simulink model "cic_filter_testing_8"  (Simulink 7.4)
settings: Solver=ode45  StartTime=0.0  StopTime=10000  RelTol=1e-3
undefined symbols (not defined in the file or in its folder): xlRetrieveParam
libraries: xbsIndex_r4 x441
(part 3 of 3)

== system cic_filter_testing_8/Parallel_CIC_filter1/Stage1_dec2/int_2/adder_tree7 ==
  sync : Inport
  din_1 : Inport  Port=2
  din_2 : Inport  Port=3
  din_3 : Inport  Port=4
  din_4 : Inport  Port=5
  din_5 : Inport  Port=6
  din_6 : Inport  Port=7
  din_7 : Inport  Port=8
  din_8 : Inport  Port=9
  adder_{0..6} (7 alike) : xbsIndex_r4/AddSub  mode=Addition  use_carryin=off  use_carryout=off  en=off  latency=1  precision=Full  arith_type=Unsigned  n_bits=18  bin_pt=17  quantization="Round  (unbiased: +/- Inf)"  overflow=Wrap  dbl_ovrd=off  use_behavioral_HDL=on  hw_selection=Fabric  pipelined=off  block_type=addsub
  sync_delay : xbsIndex_r4/Delay  en=off  latency=3  dbl_ovrd=off  reg_retiming=off  block_type=delay
      settings: block_version=11.4
  sync_out : Outport
  dout : Outport  Port=2
  wires:
  adder_6/1 -> dout/1
  adder_4/1 -> adder_6/2
  adder_5/1 -> adder_6/1
  adder_2/1 -> adder_5/2
  adder_3/1 -> adder_5/1
  adder_0/1 -> adder_4/2
  adder_1/1 -> adder_4/1
  din_7/1 -> adder_3/2
  din_8/1 -> adder_3/1
  din_5/1 -> adder_2/2
  din_6/1 -> adder_2/1
  din_3/1 -> adder_1/2
  din_4/1 -> adder_1/1
  din_1/1 -> adder_0/2
  din_2/1 -> adder_0/1
  sync_delay/1 -> sync_out/1
  sync/1 -> sync_delay/1

== system cic_filter_testing_8/Parallel_CIC_filter1/Stage1_dec2/int_2/adder_tree8 ==
  sync : Inport
  din_1 : Inport  Port=2
  din_2 : Inport  Port=3
  din_3 : Inport  Port=4
  din_4 : Inport  Port=5
  din_5 : Inport  Port=6
  din_6 : Inport  Port=7
  din_7 : Inport  Port=8
  din_8 : Inport  Port=9
  adder_{0..6} (7 alike) : xbsIndex_r4/AddSub  mode=Addition  use_carryin=off  use_carryout=off  en=off  latency=1  precision=Full  arith_type=Unsigned  n_bits=18  bin_pt=17  quantization="Round  (unbiased: +/- Inf)"  overflow=Wrap  dbl_ovrd=off  use_behavioral_HDL=on  hw_selection=Fabric  pipelined=off  block_type=addsub
  sync_delay : xbsIndex_r4/Delay  en=off  latency=3  dbl_ovrd=off  reg_retiming=off  block_type=delay
      settings: block_version=11.4
  sync_out : Outport
  dout : Outport  Port=2
  wires:
  adder_6/1 -> dout/1
  adder_4/1 -> adder_6/2
  adder_5/1 -> adder_6/1
  adder_2/1 -> adder_5/2
  adder_3/1 -> adder_5/1
  adder_0/1 -> adder_4/2
  adder_1/1 -> adder_4/1
  din_7/1 -> adder_3/2
  din_8/1 -> adder_3/1
  din_5/1 -> adder_2/2
  din_6/1 -> adder_2/1
  din_3/1 -> adder_1/2
  din_4/1 -> adder_1/1
  din_1/1 -> adder_0/2
  din_2/1 -> adder_0/1
  sync_delay/1 -> sync_out/1
  sync/1 -> sync_delay/1

== system cic_filter_testing_8/Parallel_CIC_filter1/Stage1_dec2/int_3/adder_tree1 ==
  sync : Inport
  din_1 : Inport  Port=2
  din_2 : Inport  Port=3
  din_3 : Inport  Port=4
  din_4 : Inport  Port=5
  din_5 : Inport  Port=6
  din_6 : Inport  Port=7
  din_7 : Inport  Port=8
  din_8 : Inport  Port=9
  adder_{0..6} (7 alike) : xbsIndex_r4/AddSub  mode=Addition  use_carryin=off  use_carryout=off  en=off  latency=1  precision=Full  arith_type=Unsigned  n_bits=18  bin_pt=17  quantization="Round  (unbiased: +/- Inf)"  overflow=Wrap  dbl_ovrd=off  use_behavioral_HDL=on  hw_selection=Fabric  pipelined=off  block_type=addsub
  sync_delay : xbsIndex_r4/Delay  en=off  latency=3  dbl_ovrd=off  reg_retiming=off  block_type=delay
      settings: block_version=11.4
  sync_out : Outport
  dout : Outport  Port=2
  wires:
  adder_6/1 -> dout/1
  adder_4/1 -> adder_6/2
  adder_5/1 -> adder_6/1
  adder_2/1 -> adder_5/2
  adder_3/1 -> adder_5/1
  adder_0/1 -> adder_4/2
  adder_1/1 -> adder_4/1
  din_7/1 -> adder_3/2
  din_8/1 -> adder_3/1
  din_5/1 -> adder_2/2
  din_6/1 -> adder_2/1
  din_3/1 -> adder_1/2
  din_4/1 -> adder_1/1
  din_1/1 -> adder_0/2
  din_2/1 -> adder_0/1
  sync_delay/1 -> sync_out/1
  sync/1 -> sync_delay/1

== system cic_filter_testing_8/Parallel_CIC_filter1/Stage1_dec2/int_3/adder_tree2 ==
  sync : Inport
  din_1 : Inport  Port=2
  din_2 : Inport  Port=3
  din_3 : Inport  Port=4
  din_4 : Inport  Port=5
  din_5 : Inport  Port=6
  din_6 : Inport  Port=7
  din_7 : Inport  Port=8
  din_8 : Inport  Port=9
  adder_{0..6} (7 alike) : xbsIndex_r4/AddSub  mode=Addition  use_carryin=off  use_carryout=off  en=off  latency=1  precision=Full  arith_type=Unsigned  n_bits=18  bin_pt=17  quantization="Round  (unbiased: +/- Inf)"  overflow=Wrap  dbl_ovrd=off  use_behavioral_HDL=on  hw_selection=Fabric  pipelined=off  block_type=addsub
  sync_delay : xbsIndex_r4/Delay  en=off  latency=3  dbl_ovrd=off  reg_retiming=off  block_type=delay
      settings: block_version=11.4
  sync_out : Outport
  dout : Outport  Port=2
  wires:
  adder_6/1 -> dout/1
  adder_4/1 -> adder_6/2
  adder_5/1 -> adder_6/1
  adder_2/1 -> adder_5/2
  adder_3/1 -> adder_5/1
  adder_0/1 -> adder_4/2
  adder_1/1 -> adder_4/1
  din_7/1 -> adder_3/2
  din_8/1 -> adder_3/1
  din_5/1 -> adder_2/2
  din_6/1 -> adder_2/1
  din_3/1 -> adder_1/2
  din_4/1 -> adder_1/1
  din_1/1 -> adder_0/2
  din_2/1 -> adder_0/1
  sync_delay/1 -> sync_out/1
  sync/1 -> sync_delay/1

== system cic_filter_testing_8/Parallel_CIC_filter1/Stage1_dec2/int_3/adder_tree3 ==
  sync : Inport
  din_1 : Inport  Port=2
  din_2 : Inport  Port=3
  din_3 : Inport  Port=4
  din_4 : Inport  Port=5
  din_5 : Inport  Port=6
  din_6 : Inport  Port=7
  din_7 : Inport  Port=8
  din_8 : Inport  Port=9
  adder_{0..6} (7 alike) : xbsIndex_r4/AddSub  mode=Addition  use_carryin=off  use_carryout=off  en=off  latency=1  precision=Full  arith_type=Unsigned  n_bits=18  bin_pt=17  quantization="Round  (unbiased: +/- Inf)"  overflow=Wrap  dbl_ovrd=off  use_behavioral_HDL=on  hw_selection=Fabric  pipelined=off  block_type=addsub
  sync_delay : xbsIndex_r4/Delay  en=off  latency=3  dbl_ovrd=off  reg_retiming=off  block_type=delay
      settings: block_version=11.4
  sync_out : Outport
  dout : Outport  Port=2
  wires:
  adder_6/1 -> dout/1
  adder_4/1 -> adder_6/2
  adder_5/1 -> adder_6/1
  adder_2/1 -> adder_5/2
  adder_3/1 -> adder_5/1
  adder_0/1 -> adder_4/2
  adder_1/1 -> adder_4/1
  din_7/1 -> adder_3/2
  din_8/1 -> adder_3/1
  din_5/1 -> adder_2/2
  din_6/1 -> adder_2/1
  din_3/1 -> adder_1/2
  din_4/1 -> adder_1/1
  din_1/1 -> adder_0/2
  din_2/1 -> adder_0/1
  sync_delay/1 -> sync_out/1
  sync/1 -> sync_delay/1

== system cic_filter_testing_8/Parallel_CIC_filter1/Stage1_dec2/int_3/adder_tree4 ==
  sync : Inport
  din_1 : Inport  Port=2
  din_2 : Inport  Port=3
  din_3 : Inport  Port=4
  din_4 : Inport  Port=5
  din_5 : Inport  Port=6
  din_6 : Inport  Port=7
  din_7 : Inport  Port=8
  din_8 : Inport  Port=9
  adder_{0..6} (7 alike) : xbsIndex_r4/AddSub  mode=Addition  use_carryin=off  use_carryout=off  en=off  latency=1  precision=Full  arith_type=Unsigned  n_bits=18  bin_pt=17  quantization="Round  (unbiased: +/- Inf)"  overflow=Wrap  dbl_ovrd=off  use_behavioral_HDL=on  hw_selection=Fabric  pipelined=off  block_type=addsub
  sync_delay : xbsIndex_r4/Delay  en=off  latency=3  dbl_ovrd=off  reg_retiming=off  block_type=delay
      settings: block_version=11.4
  sync_out : Outport
  dout : Outport  Port=2
  wires:
  adder_6/1 -> dout/1
  adder_4/1 -> adder_6/2
  adder_5/1 -> adder_6/1
  adder_2/1 -> adder_5/2
  adder_3/1 -> adder_5/1
  adder_0/1 -> adder_4/2
  adder_1/1 -> adder_4/1
  din_7/1 -> adder_3/2
  din_8/1 -> adder_3/1
  din_5/1 -> adder_2/2
  din_6/1 -> adder_2/1
  din_3/1 -> adder_1/2
  din_4/1 -> adder_1/1
  din_1/1 -> adder_0/2
  din_2/1 -> adder_0/1
  sync_delay/1 -> sync_out/1
  sync/1 -> sync_delay/1

== system cic_filter_testing_8/Parallel_CIC_filter1/Stage1_dec2/int_3/adder_tree5 ==
  sync : Inport
  din_1 : Inport  Port=2
  din_2 : Inport  Port=3
  din_3 : Inport  Port=4
  din_4 : Inport  Port=5
  din_5 : Inport  Port=6
  din_6 : Inport  Port=7
  din_7 : Inport  Port=8
  din_8 : Inport  Port=9
  adder_{0..6} (7 alike) : xbsIndex_r4/AddSub  mode=Addition  use_carryin=off  use_carryout=off  en=off  latency=1  precision=Full  arith_type=Unsigned  n_bits=18  bin_pt=17  quantization="Round  (unbiased: +/- Inf)"  overflow=Wrap  dbl_ovrd=off  use_behavioral_HDL=on  hw_selection=Fabric  pipelined=off  block_type=addsub
  sync_delay : xbsIndex_r4/Delay  en=off  latency=3  dbl_ovrd=off  reg_retiming=off  block_type=delay
      settings: block_version=11.4
  sync_out : Outport
  dout : Outport  Port=2
  wires:
  adder_6/1 -> dout/1
  adder_4/1 -> adder_6/2
  adder_5/1 -> adder_6/1
  adder_2/1 -> adder_5/2
  adder_3/1 -> adder_5/1
  adder_0/1 -> adder_4/2
  adder_1/1 -> adder_4/1
  din_7/1 -> adder_3/2
  din_8/1 -> adder_3/1
  din_5/1 -> adder_2/2
  din_6/1 -> adder_2/1
  din_3/1 -> adder_1/2
  din_4/1 -> adder_1/1
  din_1/1 -> adder_0/2
  din_2/1 -> adder_0/1
  sync_delay/1 -> sync_out/1
  sync/1 -> sync_delay/1

== system cic_filter_testing_8/Parallel_CIC_filter1/Stage1_dec2/int_3/adder_tree6 ==
  sync : Inport
  din_1 : Inport  Port=2
  din_2 : Inport  Port=3
  din_3 : Inport  Port=4
  din_4 : Inport  Port=5
  din_5 : Inport  Port=6
  din_6 : Inport  Port=7
  din_7 : Inport  Port=8
  din_8 : Inport  Port=9
  adder_{0..6} (7 alike) : xbsIndex_r4/AddSub  mode=Addition  use_carryin=off  use_carryout=off  en=off  latency=1  precision=Full  arith_type=Unsigned  n_bits=18  bin_pt=17  quantization="Round  (unbiased: +/- Inf)"  overflow=Wrap  dbl_ovrd=off  use_behavioral_HDL=on  hw_selection=Fabric  pipelined=off  block_type=addsub
  sync_delay : xbsIndex_r4/Delay  en=off  latency=3  dbl_ovrd=off  reg_retiming=off  block_type=delay
      settings: block_version=11.4
  sync_out : Outport
  dout : Outport  Port=2
  wires:
  adder_6/1 -> dout/1
  adder_4/1 -> adder_6/2
  adder_5/1 -> adder_6/1
  adder_2/1 -> adder_5/2
  adder_3/1 -> adder_5/1
  adder_0/1 -> adder_4/2
  adder_1/1 -> adder_4/1
  din_7/1 -> adder_3/2
  din_8/1 -> adder_3/1
  din_5/1 -> adder_2/2
  din_6/1 -> adder_2/1
  din_3/1 -> adder_1/2
  din_4/1 -> adder_1/1
  din_1/1 -> adder_0/2
  din_2/1 -> adder_0/1
  sync_delay/1 -> sync_out/1
  sync/1 -> sync_delay/1

== system cic_filter_testing_8/Parallel_CIC_filter1/Stage1_dec2/int_3/adder_tree7 ==
  sync : Inport
  din_1 : Inport  Port=2
  din_2 : Inport  Port=3
  din_3 : Inport  Port=4
  din_4 : Inport  Port=5
  din_5 : Inport  Port=6
  din_6 : Inport  Port=7
  din_7 : Inport  Port=8
  din_8 : Inport  Port=9
  adder_{0..6} (7 alike) : xbsIndex_r4/AddSub  mode=Addition  use_carryin=off  use_carryout=off  en=off  latency=1  precision=Full  arith_type=Unsigned  n_bits=18  bin_pt=17  quantization="Round  (unbiased: +/- Inf)"  overflow=Wrap  dbl_ovrd=off  use_behavioral_HDL=on  hw_selection=Fabric  pipelined=off  block_type=addsub
  sync_delay : xbsIndex_r4/Delay  en=off  latency=3  dbl_ovrd=off  reg_retiming=off  block_type=delay
      settings: block_version=11.4
  sync_out : Outport
  dout : Outport  Port=2
  wires:
  adder_6/1 -> dout/1
  adder_4/1 -> adder_6/2
  adder_5/1 -> adder_6/1
  adder_2/1 -> adder_5/2
  adder_3/1 -> adder_5/1
  adder_0/1 -> adder_4/2
  adder_1/1 -> adder_4/1
  din_7/1 -> adder_3/2
  din_8/1 -> adder_3/1
  din_5/1 -> adder_2/2
  din_6/1 -> adder_2/1
  din_3/1 -> adder_1/2
  din_4/1 -> adder_1/1
  din_1/1 -> adder_0/2
  din_2/1 -> adder_0/1
  sync_delay/1 -> sync_out/1
  sync/1 -> sync_delay/1

== system cic_filter_testing_8/Parallel_CIC_filter1/Stage1_dec2/int_3/adder_tree8 ==
  sync : Inport
  din_1 : Inport  Port=2
  din_2 : Inport  Port=3
  din_3 : Inport  Port=4
  din_4 : Inport  Port=5
  din_5 : Inport  Port=6
  din_6 : Inport  Port=7
  din_7 : Inport  Port=8
  din_8 : Inport  Port=9
  adder_{0..6} (7 alike) : xbsIndex_r4/AddSub  mode=Addition  use_carryin=off  use_carryout=off  en=off  latency=1  precision=Full  arith_type=Unsigned  n_bits=18  bin_pt=17  quantization="Round  (unbiased: +/- Inf)"  overflow=Wrap  dbl_ovrd=off  use_behavioral_HDL=on  hw_selection=Fabric  pipelined=off  block_type=addsub
  sync_delay : xbsIndex_r4/Delay  en=off  latency=3  dbl_ovrd=off  reg_retiming=off  block_type=delay
      settings: block_version=11.4
  sync_out : Outport
  dout : Outport  Port=2
  wires:
  adder_6/1 -> dout/1
  adder_4/1 -> adder_6/2
  adder_5/1 -> adder_6/1
  adder_2/1 -> adder_5/2
  adder_3/1 -> adder_5/1
  adder_0/1 -> adder_4/2
  adder_1/1 -> adder_4/1
  din_7/1 -> adder_3/2
  din_8/1 -> adder_3/1
  din_5/1 -> adder_2/2
  din_6/1 -> adder_2/1
  din_3/1 -> adder_1/2
  din_4/1 -> adder_1/1
  din_1/1 -> adder_0/2
  din_2/1 -> adder_0/1
  sync_delay/1 -> sync_out/1
  sync/1 -> sync_delay/1

== system cic_filter_testing_8/Parallel_CIC_filter1/Stage2_dec2/int_1/adder_tree1 ==
  sync : Inport
  din_1 : Inport  Port=2
  din_2 : Inport  Port=3
  din_3 : Inport  Port=4
  din_4 : Inport  Port=5
  adder_0 : xbsIndex_r4/AddSub  mode=Addition  use_carryin=off  use_carryout=off  en=off  latency=1  precision=Full  arith_type=Unsigned  n_bits=18  bin_pt=17  quantization="Round  (unbiased: +/- Inf)"  overflow=Wrap  dbl_ovrd=off  use_behavioral_HDL=on  hw_selection=Fabric  pipelined=off  block_type=addsub
  adder_1 : xbsIndex_r4/AddSub  mode=Addition  use_carryin=off  use_carryout=off  en=off  latency=1  precision=Full  arith_type=Unsigned  n_bits=18  bin_pt=17  quantization="Round  (unbiased: +/- Inf)"  overflow=Wrap  dbl_ovrd=off  use_behavioral_HDL=on  hw_selection=Fabric  pipelined=off  block_type=addsub
  adder_2 : xbsIndex_r4/AddSub  mode=Addition  use_carryin=off  use_carryout=off  en=off  latency=1  precision=Full  arith_type=Unsigned  n_bits=18  bin_pt=17  quantization="Round  (unbiased: +/- Inf)"  overflow=Wrap  dbl_ovrd=off  use_behavioral_HDL=on  hw_selection=Fabric  pipelined=off  block_type=addsub
  sync_delay : xbsIndex_r4/Delay  en=off  latency=2  dbl_ovrd=off  reg_retiming=off  block_type=delay
      settings: block_version=11.4
  sync_out : Outport
  dout : Outport  Port=2
  wires:
  adder_2/1 -> dout/1
  adder_0/1 -> adder_2/2
  adder_1/1 -> adder_2/1
  din_3/1 -> adder_1/2
  din_4/1 -> adder_1/1
  din_1/1 -> adder_0/2
  din_2/1 -> adder_0/1
  sync_delay/1 -> sync_out/1
  sync/1 -> sync_delay/1

== system cic_filter_testing_8/Parallel_CIC_filter1/Stage2_dec2/int_1/adder_tree2 ==
  sync : Inport
  din_1 : Inport  Port=2
  din_2 : Inport  Port=3
  din_3 : Inport  Port=4
  din_4 : Inport  Port=5
  adder_0 : xbsIndex_r4/AddSub  mode=Addition  use_carryin=off  use_carryout=off  en=off  latency=1  precision=Full  arith_type=Unsigned  n_bits=18  bin_pt=17  quantization="Round  (unbiased: +/- Inf)"  overflow=Wrap  dbl_ovrd=off  use_behavioral_HDL=on  hw_selection=Fabric  pipelined=off  block_type=addsub
  adder_1 : xbsIndex_r4/AddSub  mode=Addition  use_carryin=off  use_carryout=off  en=off  latency=1  precision=Full  arith_type=Unsigned  n_bits=18  bin_pt=17  quantization="Round  (unbiased: +/- Inf)"  overflow=Wrap  dbl_ovrd=off  use_behavioral_HDL=on  hw_selection=Fabric  pipelined=off  block_type=addsub
  adder_2 : xbsIndex_r4/AddSub  mode=Addition  use_carryin=off  use_carryout=off  en=off  latency=1  precision=Full  arith_type=Unsigned  n_bits=18  bin_pt=17  quantization="Round  (unbiased: +/- Inf)"  overflow=Wrap  dbl_ovrd=off  use_behavioral_HDL=on  hw_selection=Fabric  pipelined=off  block_type=addsub
  sync_delay : xbsIndex_r4/Delay  en=off  latency=2  dbl_ovrd=off  reg_retiming=off  block_type=delay
      settings: block_version=11.4
  sync_out : Outport
  dout : Outport  Port=2
  wires:
  adder_2/1 -> dout/1
  adder_0/1 -> adder_2/2
  adder_1/1 -> adder_2/1
  din_3/1 -> adder_1/2
  din_4/1 -> adder_1/1
  din_1/1 -> adder_0/2
  din_2/1 -> adder_0/1
  sync_delay/1 -> sync_out/1
  sync/1 -> sync_delay/1

== system cic_filter_testing_8/Parallel_CIC_filter1/Stage2_dec2/int_1/adder_tree3 ==
  sync : Inport
  din_1 : Inport  Port=2
  din_2 : Inport  Port=3
  din_3 : Inport  Port=4
  din_4 : Inport  Port=5
  adder_0 : xbsIndex_r4/AddSub  mode=Addition  use_carryin=off  use_carryout=off  en=off  latency=1  precision=Full  arith_type=Unsigned  n_bits=18  bin_pt=17  quantization="Round  (unbiased: +/- Inf)"  overflow=Wrap  dbl_ovrd=off  use_behavioral_HDL=on  hw_selection=Fabric  pipelined=off  block_type=addsub
  adder_1 : xbsIndex_r4/AddSub  mode=Addition  use_carryin=off  use_carryout=off  en=off  latency=1  precision=Full  arith_type=Unsigned  n_bits=18  bin_pt=17  quantization="Round  (unbiased: +/- Inf)"  overflow=Wrap  dbl_ovrd=off  use_behavioral_HDL=on  hw_selection=Fabric  pipelined=off  block_type=addsub
  adder_2 : xbsIndex_r4/AddSub  mode=Addition  use_carryin=off  use_carryout=off  en=off  latency=1  precision=Full  arith_type=Unsigned  n_bits=18  bin_pt=17  quantization="Round  (unbiased: +/- Inf)"  overflow=Wrap  dbl_ovrd=off  use_behavioral_HDL=on  hw_selection=Fabric  pipelined=off  block_type=addsub
  sync_delay : xbsIndex_r4/Delay  en=off  latency=2  dbl_ovrd=off  reg_retiming=off  block_type=delay
      settings: block_version=11.4
  sync_out : Outport
  dout : Outport  Port=2
  wires:
  adder_2/1 -> dout/1
  adder_0/1 -> adder_2/2
  adder_1/1 -> adder_2/1
  din_3/1 -> adder_1/2
  din_4/1 -> adder_1/1
  din_1/1 -> adder_0/2
  din_2/1 -> adder_0/1
  sync_delay/1 -> sync_out/1
  sync/1 -> sync_delay/1

== system cic_filter_testing_8/Parallel_CIC_filter1/Stage2_dec2/int_1/adder_tree4 ==
  sync : Inport
  din_1 : Inport  Port=2
  din_2 : Inport  Port=3
  din_3 : Inport  Port=4
  din_4 : Inport  Port=5
  adder_0 : xbsIndex_r4/AddSub  mode=Addition  use_carryin=off  use_carryout=off  en=off  latency=1  precision=Full  arith_type=Unsigned  n_bits=18  bin_pt=17  quantization="Round  (unbiased: +/- Inf)"  overflow=Wrap  dbl_ovrd=off  use_behavioral_HDL=on  hw_selection=Fabric  pipelined=off  block_type=addsub
  adder_1 : xbsIndex_r4/AddSub  mode=Addition  use_carryin=off  use_carryout=off  en=off  latency=1  precision=Full  arith_type=Unsigned  n_bits=18  bin_pt=17  quantization="Round  (unbiased: +/- Inf)"  overflow=Wrap  dbl_ovrd=off  use_behavioral_HDL=on  hw_selection=Fabric  pipelined=off  block_type=addsub
  adder_2 : xbsIndex_r4/AddSub  mode=Addition  use_carryin=off  use_carryout=off  en=off  latency=1  precision=Full  arith_type=Unsigned  n_bits=18  bin_pt=17  quantization="Round  (unbiased: +/- Inf)"  overflow=Wrap  dbl_ovrd=off  use_behavioral_HDL=on  hw_selection=Fabric  pipelined=off  block_type=addsub
  sync_delay : xbsIndex_r4/Delay  en=off  latency=2  dbl_ovrd=off  reg_retiming=off  block_type=delay
      settings: block_version=11.4
  sync_out : Outport
  dout : Outport  Port=2
  wires:
  adder_2/1 -> dout/1
  adder_0/1 -> adder_2/2
  adder_1/1 -> adder_2/1
  din_3/1 -> adder_1/2
  din_4/1 -> adder_1/1
  din_1/1 -> adder_0/2
  din_2/1 -> adder_0/1
  sync_delay/1 -> sync_out/1
  sync/1 -> sync_delay/1

== system cic_filter_testing_8/Parallel_CIC_filter1/Stage2_dec2/int_2/adder_tree1 ==
  sync : Inport
  din_1 : Inport  Port=2
  din_2 : Inport  Port=3
  din_3 : Inport  Port=4
  din_4 : Inport  Port=5
  adder_0 : xbsIndex_r4/AddSub  mode=Addition  use_carryin=off  use_carryout=off  en=off  latency=1  precision=Full  arith_type=Unsigned  n_bits=18  bin_pt=17  quantization="Round  (unbiased: +/- Inf)"  overflow=Wrap  dbl_ovrd=off  use_behavioral_HDL=on  hw_selection=Fabric  pipelined=off  block_type=addsub
  adder_1 : xbsIndex_r4/AddSub  mode=Addition  use_carryin=off  use_carryout=off  en=off  latency=1  precision=Full  arith_type=Unsigned  n_bits=18  bin_pt=17  quantization="Round  (unbiased: +/- Inf)"  overflow=Wrap  dbl_ovrd=off  use_behavioral_HDL=on  hw_selection=Fabric  pipelined=off  block_type=addsub
  adder_2 : xbsIndex_r4/AddSub  mode=Addition  use_carryin=off  use_carryout=off  en=off  latency=1  precision=Full  arith_type=Unsigned  n_bits=18  bin_pt=17  quantization="Round  (unbiased: +/- Inf)"  overflow=Wrap  dbl_ovrd=off  use_behavioral_HDL=on  hw_selection=Fabric  pipelined=off  block_type=addsub
  sync_delay : xbsIndex_r4/Delay  en=off  latency=2  dbl_ovrd=off  reg_retiming=off  block_type=delay
      settings: block_version=11.4
  sync_out : Outport
  dout : Outport  Port=2
  wires:
  adder_2/1 -> dout/1
  adder_0/1 -> adder_2/2
  adder_1/1 -> adder_2/1
  din_3/1 -> adder_1/2
  din_4/1 -> adder_1/1
  din_1/1 -> adder_0/2
  din_2/1 -> adder_0/1
  sync_delay/1 -> sync_out/1
  sync/1 -> sync_delay/1

== system cic_filter_testing_8/Parallel_CIC_filter1/Stage2_dec2/int_2/adder_tree2 ==
  sync : Inport
  din_1 : Inport  Port=2
  din_2 : Inport  Port=3
  din_3 : Inport  Port=4
  din_4 : Inport  Port=5
  adder_0 : xbsIndex_r4/AddSub  mode=Addition  use_carryin=off  use_carryout=off  en=off  latency=1  precision=Full  arith_type=Unsigned  n_bits=18  bin_pt=17  quantization="Round  (unbiased: +/- Inf)"  overflow=Wrap  dbl_ovrd=off  use_behavioral_HDL=on  hw_selection=Fabric  pipelined=off  block_type=addsub
  adder_1 : xbsIndex_r4/AddSub  mode=Addition  use_carryin=off  use_carryout=off  en=off  latency=1  precision=Full  arith_type=Unsigned  n_bits=18  bin_pt=17  quantization="Round  (unbiased: +/- Inf)"  overflow=Wrap  dbl_ovrd=off  use_behavioral_HDL=on  hw_selection=Fabric  pipelined=off  block_type=addsub
  adder_2 : xbsIndex_r4/AddSub  mode=Addition  use_carryin=off  use_carryout=off  en=off  latency=1  precision=Full  arith_type=Unsigned  n_bits=18  bin_pt=17  quantization="Round  (unbiased: +/- Inf)"  overflow=Wrap  dbl_ovrd=off  use_behavioral_HDL=on  hw_selection=Fabric  pipelined=off  block_type=addsub
  sync_delay : xbsIndex_r4/Delay  en=off  latency=2  dbl_ovrd=off  reg_retiming=off  block_type=delay
      settings: block_version=11.4
  sync_out : Outport
  dout : Outport  Port=2
  wires:
  adder_2/1 -> dout/1
  adder_0/1 -> adder_2/2
  adder_1/1 -> adder_2/1
  din_3/1 -> adder_1/2
  din_4/1 -> adder_1/1
  din_1/1 -> adder_0/2
  din_2/1 -> adder_0/1
  sync_delay/1 -> sync_out/1
  sync/1 -> sync_delay/1

== system cic_filter_testing_8/Parallel_CIC_filter1/Stage2_dec2/int_2/adder_tree3 ==
  sync : Inport
  din_1 : Inport  Port=2
  din_2 : Inport  Port=3
  din_3 : Inport  Port=4
  din_4 : Inport  Port=5
  adder_0 : xbsIndex_r4/AddSub  mode=Addition  use_carryin=off  use_carryout=off  en=off  latency=1  precision=Full  arith_type=Unsigned  n_bits=18  bin_pt=17  quantization="Round  (unbiased: +/- Inf)"  overflow=Wrap  dbl_ovrd=off  use_behavioral_HDL=on  hw_selection=Fabric  pipelined=off  block_type=addsub
  adder_1 : xbsIndex_r4/AddSub  mode=Addition  use_carryin=off  use_carryout=off  en=off  latency=1  precision=Full  arith_type=Unsigned  n_bits=18  bin_pt=17  quantization="Round  (unbiased: +/- Inf)"  overflow=Wrap  dbl_ovrd=off  use_behavioral_HDL=on  hw_selection=Fabric  pipelined=off  block_type=addsub
  adder_2 : xbsIndex_r4/AddSub  mode=Addition  use_carryin=off  use_carryout=off  en=off  latency=1  precision=Full  arith_type=Unsigned  n_bits=18  bin_pt=17  quantization="Round  (unbiased: +/- Inf)"  overflow=Wrap  dbl_ovrd=off  use_behavioral_HDL=on  hw_selection=Fabric  pipelined=off  block_type=addsub
  sync_delay : xbsIndex_r4/Delay  en=off  latency=2  dbl_ovrd=off  reg_retiming=off  block_type=delay
      settings: block_version=11.4
  sync_out : Outport
  dout : Outport  Port=2
  wires:
  adder_2/1 -> dout/1
  adder_0/1 -> adder_2/2
  adder_1/1 -> adder_2/1
  din_3/1 -> adder_1/2
  din_4/1 -> adder_1/1
  din_1/1 -> adder_0/2
  din_2/1 -> adder_0/1
  sync_delay/1 -> sync_out/1
  sync/1 -> sync_delay/1

== system cic_filter_testing_8/Parallel_CIC_filter1/Stage2_dec2/int_2/adder_tree4 ==
  sync : Inport
  din_1 : Inport  Port=2
  din_2 : Inport  Port=3
  din_3 : Inport  Port=4
  din_4 : Inport  Port=5
  adder_0 : xbsIndex_r4/AddSub  mode=Addition  use_carryin=off  use_carryout=off  en=off  latency=1  precision=Full  arith_type=Unsigned  n_bits=18  bin_pt=17  quantization="Round  (unbiased: +/- Inf)"  overflow=Wrap  dbl_ovrd=off  use_behavioral_HDL=on  hw_selection=Fabric  pipelined=off  block_type=addsub
  adder_1 : xbsIndex_r4/AddSub  mode=Addition  use_carryin=off  use_carryout=off  en=off  latency=1  precision=Full  arith_type=Unsigned  n_bits=18  bin_pt=17  quantization="Round  (unbiased: +/- Inf)"  overflow=Wrap  dbl_ovrd=off  use_behavioral_HDL=on  hw_selection=Fabric  pipelined=off  block_type=addsub
  adder_2 : xbsIndex_r4/AddSub  mode=Addition  use_carryin=off  use_carryout=off  en=off  latency=1  precision=Full  arith_type=Unsigned  n_bits=18  bin_pt=17  quantization="Round  (unbiased: +/- Inf)"  overflow=Wrap  dbl_ovrd=off  use_behavioral_HDL=on  hw_selection=Fabric  pipelined=off  block_type=addsub
  sync_delay : xbsIndex_r4/Delay  en=off  latency=2  dbl_ovrd=off  reg_retiming=off  block_type=delay
      settings: block_version=11.4
  sync_out : Outport
  dout : Outport  Port=2
  wires:
  adder_2/1 -> dout/1
  adder_0/1 -> adder_2/2
  adder_1/1 -> adder_2/1
  din_3/1 -> adder_1/2
  din_4/1 -> adder_1/1
  din_1/1 -> adder_0/2
  din_2/1 -> adder_0/1
  sync_delay/1 -> sync_out/1
  sync/1 -> sync_delay/1

== system cic_filter_testing_8/Parallel_CIC_filter1/Stage2_dec2/int_3/adder_tree1 ==
  sync : Inport
  din_1 : Inport  Port=2
  din_2 : Inport  Port=3
  din_3 : Inport  Port=4
  din_4 : Inport  Port=5
  adder_0 : xbsIndex_r4/AddSub  mode=Addition  use_carryin=off  use_carryout=off  en=off  latency=1  precision=Full  arith_type=Unsigned  n_bits=18  bin_pt=17  quantization="Round  (unbiased: +/- Inf)"  overflow=Wrap  dbl_ovrd=off  use_behavioral_HDL=on  hw_selection=Fabric  pipelined=off  block_type=addsub
  adder_1 : xbsIndex_r4/AddSub  mode=Addition  use_carryin=off  use_carryout=off  en=off  latency=1  precision=Full  arith_type=Unsigned  n_bits=18  bin_pt=17  quantization="Round  (unbiased: +/- Inf)"  overflow=Wrap  dbl_ovrd=off  use_behavioral_HDL=on  hw_selection=Fabric  pipelined=off  block_type=addsub
  adder_2 : xbsIndex_r4/AddSub  mode=Addition  use_carryin=off  use_carryout=off  en=off  latency=1  precision=Full  arith_type=Unsigned  n_bits=18  bin_pt=17  quantization="Round  (unbiased: +/- Inf)"  overflow=Wrap  dbl_ovrd=off  use_behavioral_HDL=on  hw_selection=Fabric  pipelined=off  block_type=addsub
  sync_delay : xbsIndex_r4/Delay  en=off  latency=2  dbl_ovrd=off  reg_retiming=off  block_type=delay
      settings: block_version=11.4
  sync_out : Outport
  dout : Outport  Port=2
  wires:
  adder_2/1 -> dout/1
  adder_0/1 -> adder_2/2
  adder_1/1 -> adder_2/1
  din_3/1 -> adder_1/2
  din_4/1 -> adder_1/1
  din_1/1 -> adder_0/2
  din_2/1 -> adder_0/1
  sync_delay/1 -> sync_out/1
  sync/1 -> sync_delay/1

== system cic_filter_testing_8/Parallel_CIC_filter1/Stage2_dec2/int_3/adder_tree2 ==
  sync : Inport
  din_1 : Inport  Port=2
  din_2 : Inport  Port=3
  din_3 : Inport  Port=4
  din_4 : Inport  Port=5
  adder_0 : xbsIndex_r4/AddSub  mode=Addition  use_carryin=off  use_carryout=off  en=off  latency=1  precision=Full  arith_type=Unsigned  n_bits=18  bin_pt=17  quantization="Round  (unbiased: +/- Inf)"  overflow=Wrap  dbl_ovrd=off  use_behavioral_HDL=on  hw_selection=Fabric  pipelined=off  block_type=addsub
  adder_1 : xbsIndex_r4/AddSub  mode=Addition  use_carryin=off  use_carryout=off  en=off  latency=1  precision=Full  arith_type=Unsigned  n_bits=18  bin_pt=17  quantization="Round  (unbiased: +/- Inf)"  overflow=Wrap  dbl_ovrd=off  use_behavioral_HDL=on  hw_selection=Fabric  pipelined=off  block_type=addsub
  adder_2 : xbsIndex_r4/AddSub  mode=Addition  use_carryin=off  use_carryout=off  en=off  latency=1  precision=Full  arith_type=Unsigned  n_bits=18  bin_pt=17  quantization="Round  (unbiased: +/- Inf)"  overflow=Wrap  dbl_ovrd=off  use_behavioral_HDL=on  hw_selection=Fabric  pipelined=off  block_type=addsub
  sync_delay : xbsIndex_r4/Delay  en=off  latency=2  dbl_ovrd=off  reg_retiming=off  block_type=delay
      settings: block_version=11.4
  sync_out : Outport
  dout : Outport  Port=2
  wires:
  adder_2/1 -> dout/1
  adder_0/1 -> adder_2/2
  adder_1/1 -> adder_2/1
  din_3/1 -> adder_1/2
  din_4/1 -> adder_1/1
  din_1/1 -> adder_0/2
  din_2/1 -> adder_0/1
  sync_delay/1 -> sync_out/1
  sync/1 -> sync_delay/1

== system cic_filter_testing_8/Parallel_CIC_filter1/Stage2_dec2/int_3/adder_tree3 ==
  sync : Inport
  din_1 : Inport  Port=2
  din_2 : Inport  Port=3
  din_3 : Inport  Port=4
  din_4 : Inport  Port=5
  adder_0 : xbsIndex_r4/AddSub  mode=Addition  use_carryin=off  use_carryout=off  en=off  latency=1  precision=Full  arith_type=Unsigned  n_bits=18  bin_pt=17  quantization="Round  (unbiased: +/- Inf)"  overflow=Wrap  dbl_ovrd=off  use_behavioral_HDL=on  hw_selection=Fabric  pipelined=off  block_type=addsub
  adder_1 : xbsIndex_r4/AddSub  mode=Addition  use_carryin=off  use_carryout=off  en=off  latency=1  precision=Full  arith_type=Unsigned  n_bits=18  bin_pt=17  quantization="Round  (unbiased: +/- Inf)"  overflow=Wrap  dbl_ovrd=off  use_behavioral_HDL=on  hw_selection=Fabric  pipelined=off  block_type=addsub
  adder_2 : xbsIndex_r4/AddSub  mode=Addition  use_carryin=off  use_carryout=off  en=off  latency=1  precision=Full  arith_type=Unsigned  n_bits=18  bin_pt=17  quantization="Round  (unbiased: +/- Inf)"  overflow=Wrap  dbl_ovrd=off  use_behavioral_HDL=on  hw_selection=Fabric  pipelined=off  block_type=addsub
  sync_delay : xbsIndex_r4/Delay  en=off  latency=2  dbl_ovrd=off  reg_retiming=off  block_type=delay
      settings: block_version=11.4
  sync_out : Outport
  dout : Outport  Port=2
  wires:
  adder_2/1 -> dout/1
  adder_0/1 -> adder_2/2
  adder_1/1 -> adder_2/1
  din_3/1 -> adder_1/2
  din_4/1 -> adder_1/1
  din_1/1 -> adder_0/2
  din_2/1 -> adder_0/1
  sync_delay/1 -> sync_out/1
  sync/1 -> sync_delay/1

== system cic_filter_testing_8/Parallel_CIC_filter1/Stage2_dec2/int_3/adder_tree4 ==
  sync : Inport
  din_1 : Inport  Port=2
  din_2 : Inport  Port=3
  din_3 : Inport  Port=4
  din_4 : Inport  Port=5
  adder_0 : xbsIndex_r4/AddSub  mode=Addition  use_carryin=off  use_carryout=off  en=off  latency=1  precision=Full  arith_type=Unsigned  n_bits=18  bin_pt=17  quantization="Round  (unbiased: +/- Inf)"  overflow=Wrap  dbl_ovrd=off  use_behavioral_HDL=on  hw_selection=Fabric  pipelined=off  block_type=addsub
  adder_1 : xbsIndex_r4/AddSub  mode=Addition  use_carryin=off  use_carryout=off  en=off  latency=1  precision=Full  arith_type=Unsigned  n_bits=18  bin_pt=17  quantization="Round  (unbiased: +/- Inf)"  overflow=Wrap  dbl_ovrd=off  use_behavioral_HDL=on  hw_selection=Fabric  pipelined=off  block_type=addsub
  adder_2 : xbsIndex_r4/AddSub  mode=Addition  use_carryin=off  use_carryout=off  en=off  latency=1  precision=Full  arith_type=Unsigned  n_bits=18  bin_pt=17  quantization="Round  (unbiased: +/- Inf)"  overflow=Wrap  dbl_ovrd=off  use_behavioral_HDL=on  hw_selection=Fabric  pipelined=off  block_type=addsub
  sync_delay : xbsIndex_r4/Delay  en=off  latency=2  dbl_ovrd=off  reg_retiming=off  block_type=delay
      settings: block_version=11.4
  sync_out : Outport
  dout : Outport  Port=2
  wires:
  adder_2/1 -> dout/1
  adder_0/1 -> adder_2/2
  adder_1/1 -> adder_2/1
  din_3/1 -> adder_1/2
  din_4/1 -> adder_1/1
  din_1/1 -> adder_0/2
  din_2/1 -> adder_0/1
  sync_delay/1 -> sync_out/1
  sync/1 -> sync_delay/1

== system cic_filter_testing_8/Parallel_CIC_filter1/Stage3_dec2/int_1/adder_tree1 ==
  sync : Inport
  din_1 : Inport  Port=2
  din_2 : Inport  Port=3
  adder_0 : xbsIndex_r4/AddSub  mode=Addition  use_carryin=off  use_carryout=off  en=off  latency=1  precision=Full  arith_type=Unsigned  n_bits=18  bin_pt=17  quantization="Round  (unbiased: +/- Inf)"  overflow=Wrap  dbl_ovrd=off  use_behavioral_HDL=on  hw_selection=Fabric  pipelined=off  block_type=addsub
  sync_delay : xbsIndex_r4/Delay  en=off  latency=1  dbl_ovrd=off  reg_retiming=off  block_type=delay
      settings: block_version=11.4
  sync_out : Outport
  dout : Outport  Port=2
  wires:
  adder_0/1 -> dout/1
  din_1/1 -> adder_0/2
  din_2/1 -> adder_0/1
  sync_delay/1 -> sync_out/1
  sync/1 -> sync_delay/1

== system cic_filter_testing_8/Parallel_CIC_filter1/Stage3_dec2/int_1/adder_tree2 ==
  sync : Inport
  din_1 : Inport  Port=2
  din_2 : Inport  Port=3
  adder_0 : xbsIndex_r4/AddSub  mode=Addition  use_carryin=off  use_carryout=off  en=off  latency=1  precision=Full  arith_type=Unsigned  n_bits=18  bin_pt=17  quantization="Round  (unbiased: +/- Inf)"  overflow=Wrap  dbl_ovrd=off  use_behavioral_HDL=on  hw_selection=Fabric  pipelined=off  block_type=addsub
  sync_delay : xbsIndex_r4/Delay  en=off  latency=1  dbl_ovrd=off  reg_retiming=off  block_type=delay
      settings: block_version=11.4
  sync_out : Outport
  dout : Outport  Port=2
  wires:
  adder_0/1 -> dout/1
  din_1/1 -> adder_0/2
  din_2/1 -> adder_0/1
  sync_delay/1 -> sync_out/1
  sync/1 -> sync_delay/1

== system cic_filter_testing_8/Parallel_CIC_filter1/Stage3_dec2/int_2/adder_tree1 ==
  sync : Inport
  din_1 : Inport  Port=2
  din_2 : Inport  Port=3
  adder_0 : xbsIndex_r4/AddSub  mode=Addition  use_carryin=off  use_carryout=off  en=off  latency=1  precision=Full  arith_type=Unsigned  n_bits=18  bin_pt=17  quantization="Round  (unbiased: +/- Inf)"  overflow=Wrap  dbl_ovrd=off  use_behavioral_HDL=on  hw_selection=Fabric  pipelined=off  block_type=addsub
  sync_delay : xbsIndex_r4/Delay  en=off  latency=1  dbl_ovrd=off  reg_retiming=off  block_type=delay
      settings: block_version=11.4
  sync_out : Outport
  dout : Outport  Port=2
  wires:
  adder_0/1 -> dout/1
  din_1/1 -> adder_0/2
  din_2/1 -> adder_0/1
  sync_delay/1 -> sync_out/1
  sync/1 -> sync_delay/1

== system cic_filter_testing_8/Parallel_CIC_filter1/Stage3_dec2/int_2/adder_tree2 ==
  sync : Inport
  din_1 : Inport  Port=2
  din_2 : Inport  Port=3
  adder_0 : xbsIndex_r4/AddSub  mode=Addition  use_carryin=off  use_carryout=off  en=off  latency=1  precision=Full  arith_type=Unsigned  n_bits=18  bin_pt=17  quantization="Round  (unbiased: +/- Inf)"  overflow=Wrap  dbl_ovrd=off  use_behavioral_HDL=on  hw_selection=Fabric  pipelined=off  block_type=addsub
  sync_delay : xbsIndex_r4/Delay  en=off  latency=1  dbl_ovrd=off  reg_retiming=off  block_type=delay
      settings: block_version=11.4
  sync_out : Outport
  dout : Outport  Port=2
  wires:
  adder_0/1 -> dout/1
  din_1/1 -> adder_0/2
  din_2/1 -> adder_0/1
  sync_delay/1 -> sync_out/1
  sync/1 -> sync_delay/1

== system cic_filter_testing_8/Parallel_CIC_filter1/Stage3_dec2/int_3/adder_tree1 ==
  sync : Inport
  din_1 : Inport  Port=2
  din_2 : Inport  Port=3
  adder_0 : xbsIndex_r4/AddSub  mode=Addition  use_carryin=off  use_carryout=off  en=off  latency=1  precision=Full  arith_type=Unsigned  n_bits=18  bin_pt=17  quantization="Round  (unbiased: +/- Inf)"  overflow=Wrap  dbl_ovrd=off  use_behavioral_HDL=on  hw_selection=Fabric  pipelined=off  block_type=addsub
  sync_delay : xbsIndex_r4/Delay  en=off  latency=1  dbl_ovrd=off  reg_retiming=off  block_type=delay
      settings: block_version=11.4
  sync_out : Outport
  dout : Outport  Port=2
  wires:
  adder_0/1 -> dout/1
  din_1/1 -> adder_0/2
  din_2/1 -> adder_0/1
  sync_delay/1 -> sync_out/1
  sync/1 -> sync_delay/1

== system cic_filter_testing_8/Parallel_CIC_filter1/Stage3_dec2/int_3/adder_tree2 ==
  sync : Inport
  din_1 : Inport  Port=2
  din_2 : Inport  Port=3
  adder_0 : xbsIndex_r4/AddSub  mode=Addition  use_carryin=off  use_carryout=off  en=off  latency=1  precision=Full  arith_type=Unsigned  n_bits=18  bin_pt=17  quantization="Round  (unbiased: +/- Inf)"  overflow=Wrap  dbl_ovrd=off  use_behavioral_HDL=on  hw_selection=Fabric  pipelined=off  block_type=addsub
  sync_delay : xbsIndex_r4/Delay  en=off  latency=1  dbl_ovrd=off  reg_retiming=off  block_type=delay
      settings: block_version=11.4
  sync_out : Outport
  dout : Outport  Port=2
  wires:
  adder_0/1 -> dout/1
  din_1/1 -> adder_0/2
  din_2/1 -> adder_0/1
  sync_delay/1 -> sync_out/1
  sync/1 -> sync_delay/1
